simulink model "step_response"  (R2022a)
settings: Solver=VariableStepAuto  StartTime=0.0  StopTime=1000.0  RelTol=1e-3
settings Model: Creator=SPY  LastModifiedBy=SPY

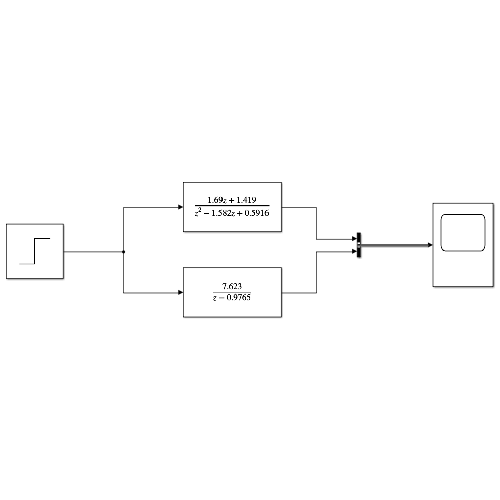
[thumbnail: Simulink's stored preview of the top-level diagram]
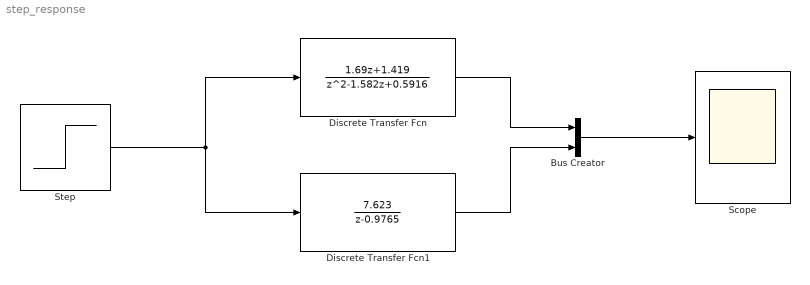
== system step_response ==
  Bus Creator : BusCreator  Inputs=2
  Discrete Transfer Fcn : DiscreteTransferFcn  Numerator=[1.69 1.419]  Denominator=[1 -1.582 0.5916]
  Discrete Transfer Fcn1 : DiscreteTransferFcn  Numerator=[7.623]  Denominator=[1 -0.9765]
  Scope : Scope
  Step : Step  SampleTime=5
  wires:
  Step/1 -> Discrete Transfer Fcn/1, Discrete Transfer Fcn1/1
  Discrete Transfer Fcn/1 -> Bus Creator/1
  Discrete Transfer Fcn1/1 -> Bus Creator/2
  Bus Creator/1 -> Scope/1
